simulink library "libbha_parameters"  (R2015b)
settings: Solver=FixedStepDiscrete  StartTime=0.0  StopTime=Inf  FixedStep=0.004  RelTol=1e-3
PostLoadFcn:
  | , if any(exist('dsrtsu_mdlpostloadfcn', 'file') == [2, 3, 6]), try dsrtsu_mdlpostloadfcn('Execute', bdroot); catch fprintf('Error in PostLoadFcn (dsrtsu_mdlpostloadfcn) for model "%s":\n %s\n', bdroot, lasterr); end, end,
undefined symbols (not defined in the file or in its folder): BHA, CONST
libraries: libbha_kinematic x12
(part 1 of 2)
settings Model: DSRTSU_INTERNAL_RTI_VER=470  DSRTSU_INTERNAL_RTI_TYPE=rti1005  DSRTSU_INTERNAL_RTIFPGA=60  Creator=Falkenhahn  LastModifiedBy=fav
settings DataIOCC: SaveFormat=Array
settings OptimizationCC: BlockReduction=off  OptimizeBlockIOStorage=off  BufferReuse=off  GlobalBufferReuse=off  ExpressionFolding=off  LocalBlockOutputs=off
settings DebuggingCC: UnderspecifiedInitializationDetection=Classic  MergeDetectMultiDrivingBlocksExec=none  SolverPrmCheckMsg=warning
settings HardwareCC: ProdBitPerPointer=32  ProdLargestAtomicFloat=None  ProdEndianess=BigEndian  ProdWordSize=32  ProdHWDeviceType=Generic->Custom  TargetIntDivRoundTo=Zero  TargetEndianess=BigEndian  TargetHWDeviceType=Generic->Custom
settings RTWCC: SystemTargetFile=rti1007.tlc  MakeCommand=make_rti  TemplateMakefile=rti1007.tmf  Description=dSPACE DS1007 Hardware Platform
settings STFCustomTargetCC: ParMdlRefBuildCompliant=on  ConcurrentExecutionCompliant=off  MatFileLogging=on  SystemTargetFile=rti1007.tlc
settings GRTTargetCC: CompOptLevelCompliant=off  ConcurrentExecutionCompliant=off  GeneratePreprocessorConditionals=Disable all  CombineOutputUpdateFcns=off  GRTInterface=on  UseToolchainInfoCompliant=off  ExtModeMexFile=noextcomm
settings ConfigComp: CovModelRefEnable=Off

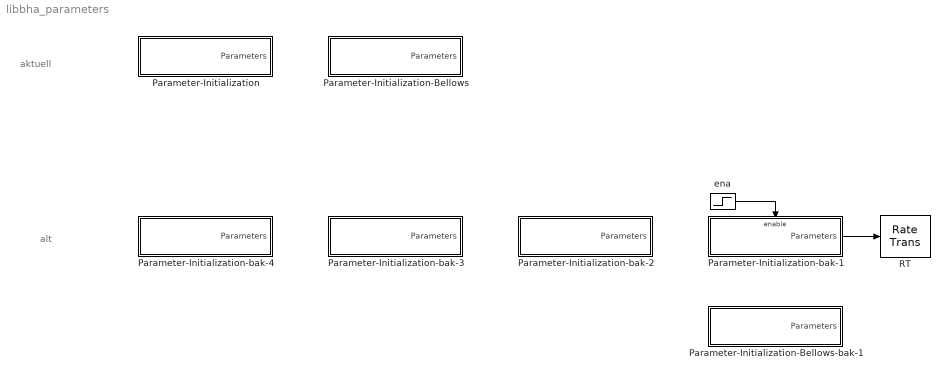
== system libbha_parameters ==
  note: aktuell
  note: alt
  Parameter-Initialization : Subsystem  mask{bha_var_choice=BHA, tA=CONST.tA}
      mask prompts: bha_var_choice "BHA-Parameter"; tA "sample time"
      mask init:
      | if bha_var_choice == 1 % BHA
      |     bha_var = evalin('base','BHA');
      | elseif bha_var_choice == 2 % BHASIM
      |     bha_var = evalin('base','BHASIM');
      | else % default: BHA
      |     bha_var = evalin('base','BHA');
      | end
      settings: AttributesFormatString=|
      | BHA-Variable: %<bha_var_choice>
      | sample time: %<tA>
      mask TypeOptions bha_var_choice: BHA | BHASIM
  Parameter-Initialization-Bellows : Subsystem  mask{bha_var_choice=BHA, tA=CONST.tA}
      mask prompts: bha_var_choice "BHA-Parameter"; tA "sample time"
      mask init:
      | if bha_var_choice == 1 % BHA
      |     bha_var = evalin('base','BHA');
      | elseif bha_var_choice == 2 % BHASIM
      |     bha_var = evalin('base','BHASIM');
      | else % default: BHA
      |     bha_var = evalin('base','BHA');
      | end
      settings: AttributesFormatString=|
      | BHA-Variable: %<bha_var_choice>\nsample time: %<tA>
      | (ohne Manipulatordaten)
      mask TypeOptions bha_var_choice: BHA | BHASIM
  Parameter-Initialization-Bellows-bak-1 : Subsystem  mask{bha_var_choice=BHA, tA=CONST.tA}
      mask prompts: bha_var_choice "BHA-Parameter"; tA "sample time"
      mask init:
      | if bha_var_choice == 1 % BHA
      |     bha_var = evalin('base','BHA');
      | elseif bha_var_choice == 2 % BHASIM
      |     bha_var = evalin('base','BHASIM');
      | else % default: BHA
      |     bha_var = evalin('base','BHA');
      | end
      settings: AttributesFormatString=|
      | BHA-Variable: %<bha_var_choice>\nsample time: %<tA>
      | (ohne Manipulatordaten)
      mask TypeOptions bha_var_choice: BHA | BHASIM
  Parameter-Initialization-bak-1 : Subsystem  mask{bha_var_choice=BHA}
      mask prompts: bha_var_choice "BHA-Parameter"
      mask init:
      | if bha_var_choice == 1 % BHA
      |     bha_var = evalin('base','BHA');
      | elseif bha_var_choice == 2 % BHASIM
      |     bha_var = evalin('base','BHASIM');
      | else % default: BHA
      |     bha_var = evalin('base','BHA');
      | end
      settings: AttributesFormatString=BHA-Variable: %<bha_var_choice>
      mask TypeOptions bha_var_choice: BHA | BHASIM
  Parameter-Initialization-bak-2 : Subsystem  mask{bha_var_choice=BHA, tA=CONST.tA}
      mask prompts: bha_var_choice "BHA-Parameter"; tA "sample time"
      mask init:
      | if bha_var_choice == 1 % BHA
      |     bha_var = evalin('base','BHA');
      | elseif bha_var_choice == 2 % BHASIM
      |     bha_var = evalin('base','BHASIM');
      | else % default: BHA
      |     bha_var = evalin('base','BHA');
      | end
      settings: AttributesFormatString=BHA-Variable: %<bha_var_choice>\nsample time: %<tA>
      mask TypeOptions bha_var_choice: BHA | BHASIM
  Parameter-Initialization-bak-3 : Subsystem  mask{bha_var_choice=BHA, tA=CONST.tA}
      mask prompts: bha_var_choice "BHA-Parameter"; tA "sample time"
      mask init:
      | if bha_var_choice == 1 % BHA
      |     bha_var = evalin('base','BHA');
      | elseif bha_var_choice == 2 % BHASIM
      |     bha_var = evalin('base','BHASIM');
      | else % default: BHA
      |     bha_var = evalin('base','BHA');
      | end
      settings: AttributesFormatString=BHA-Variable: %<bha_var_choice>\nsample time: %<tA>
      mask TypeOptions bha_var_choice: BHA | BHASIM
  Parameter-Initialization-bak-4 : Subsystem  mask{bha_var_choice=BHA, tA=CONST.tA}
      mask prompts: bha_var_choice "BHA-Parameter"; tA "sample time"
      mask init:
      | if bha_var_choice == 1 % BHA
      |     bha_var = evalin('base','BHA');
      | elseif bha_var_choice == 2 % BHASIM
      |     bha_var = evalin('base','BHASIM');
      | else % default: BHA
      |     bha_var = evalin('base','BHA');
      | end
      settings: AttributesFormatString=BHA-Variable: %<bha_var_choice>\nsample time: %<tA>
      mask TypeOptions bha_var_choice: BHA | BHASIM
  RT : RateTransition  Deterministic=off  OutPortSampleTime=CTRL.tA.obsv_pr
      settings: AttributesFormatString=%<OutPortSampleTime>
  ena : Step  Time=2*CONST.tA  Before=1  After=0  SampleTime=CONST.tA
  wires:
  ena/1 -> Parameter-Initialization-bak-1/Enable
  Parameter-Initialization-bak-1/1(Parameters) -> RT/1

== system libbha_parameters/Parameter-Initialization ==
  Calculate Parameters Once : Subsystem
  ena : Step  Time=2*tA  Before=1  After=0  SampleTime=tA
  Parameters : Outport  SourceOfInitialOutputValue=Input signal
  wires:
  Calculate Parameters Once/1(Parameters) -> Parameters/1
  ena/1 -> Calculate Parameters Once/Enable

== system libbha_parameters/Parameter-Initialization-Bellows ==
  Calculate Parameters Once : Subsystem
  ena : Step  Time=2*tA  Before=1  After=0  SampleTime=tA
  Parameters : Outport  SourceOfInitialOutputValue=Input signal
  wires:
  ena/1 -> Calculate Parameters Once/Enable
  Calculate Parameters Once/1(Parameters) -> Parameters/1

== system libbha_parameters/Parameter-Initialization-Bellows-bak-1 ==
  Calculate Parameters Once : Subsystem
  ena : Step  Time=2*tA  Before=1  After=0  SampleTime=tA
  Parameters : Outport  SourceOfInitialOutputValue=Input signal
  wires:
  Calculate Parameters Once/1(Parameters) -> Parameters/1
  ena/1 -> Calculate Parameters Once/Enable

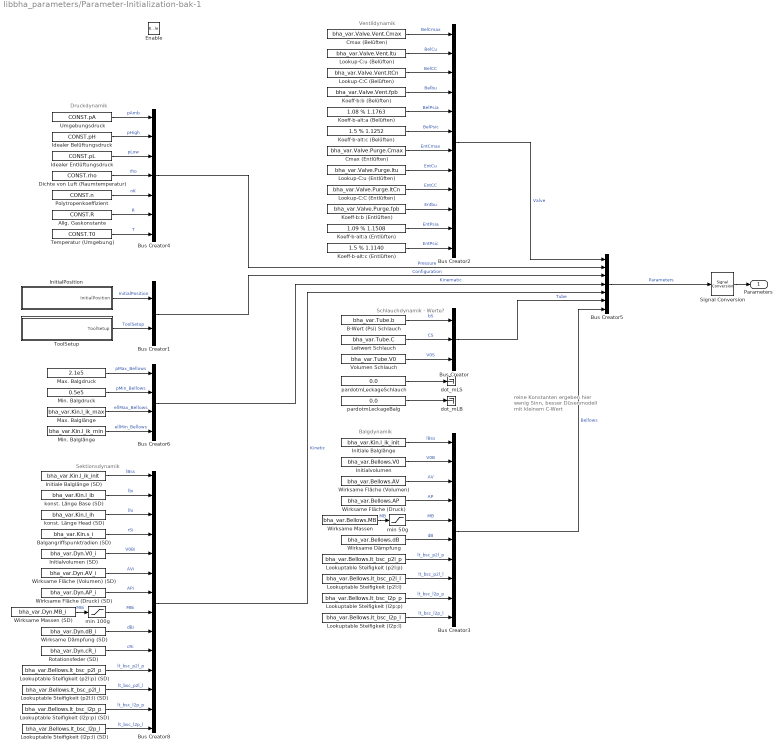
== system libbha_parameters/Parameter-Initialization-bak-1 ==
  note: Sektionsdynamik
  note: Ventildynamik
  note: Druckdynamik
  note: Balgdynamik
  note: Schlauchdynamik - Werte?
  note: reine Konstanten ergeben
      | hier wenig Sinn, besser
      | Düsenmodell mit kleinem C-Wert
  Enable : EnablePort  PropagateVarSize=During execution
  Allg. Gaskonstante : Constant  Value=CONST.R
  B-Wert (Psi) Schlauch : Constant  Value=bha_var.Tube.b
  Balgangriffspunktradien (SD) : Constant  Value=bha_var.Kin.s_i
  Bus Creator1 : BusCreator  Inputs=2
  Bus Creator3 : BusCreator  Inputs=10
  Bus Creator4 : BusCreator  Inputs=7
  Bus Creator6 : BusCreator  Inputs=4
  Bus Creator8 : BusCreator  Inputs=14
  Bus Creator : BusCreator  Inputs=3
  Bus Creator2 : BusCreator  Inputs=12
  Bus Creator5 : BusCreator  Inputs=7
  Cmax (Belüften) : Constant  Value=bha_var.Valve.Vent.Cmax
  Cmax (Entlüften) : Constant  Value=bha_var.Valve.Purge.Cmax
  Dichte von Luft (Raumtemperatur) : Constant  Value=CONST.rho
  Idealer Belüftungsdruck : Constant  Value=CONST.pH
  Idealer Entlüftungsdruck : Constant  Value=CONST.pL
  InitialPosition : Subsystem
  Initiale Balglänge : Constant  Value=bha_var.Kin.l_ik_init
  Initiale Balglänge (SD) : Constant  Value=bha_var.Kin.l_ik_init
  Initialvolumen : Constant  Value=bha_var.Bellows.V0
  Initialvolumen (SD) : Constant  Value=bha_var.Dyn.V0_i
  Koeff-b-alt:a (Belüften) : Constant  Value=1.08 % 1.1763
  Koeff-b-alt:a (Entlüften) : Constant  Value=1.09 % 1.1508
  Koeff-b-alt:c (Belüften) : Constant  Value=1.5 % 1.1252
  Koeff-b-alt:c (Entlüften) : Constant  Value=1.5 % 1.1140
  Koeff-b:b (Belüften) : Constant  Value=bha_var.Valve.Vent.fpb
  Koeff-b:b (Entlüften) : Constant  Value=bha_var.Valve.Purge.fpb
  Leitwert Schlauch : Constant  Value=bha_var.Tube.C
  Lookup-C:C (Belüften) : Constant  Value=bha_var.Valve.Vent.ltCn
  Lookup-C:C (Entlüften) : Constant  Value=bha_var.Valve.Purge.ltCn
  Lookup-C:u (Belüften) : Constant  Value=bha_var.Valve.Vent.ltu
  Lookup-C:u (Entlüften) : Constant  Value=bha_var.Valve.Purge.ltu
  Lookuptable Steifigkeit (l2p:l) : Constant  Value=bha_var.Bellows.lt_bsc_l2p_l
  Lookuptable Steifigkeit (l2p:l) (SD) : Constant  Value=bha_var.Bellows.lt_bsc_l2p_l
  Lookuptable Steifigkeit (l2p:p) : Constant  Value=bha_var.Bellows.lt_bsc_l2p_p
  Lookuptable Steifigkeit (l2p:p) (SD) : Constant  Value=bha_var.Bellows.lt_bsc_l2p_p
  Lookuptable Steifigkeit (p2l:l) : Constant  Value=bha_var.Bellows.lt_bsc_p2l_l
  Lookuptable Steifigkeit (p2l:l) (SD) : Constant  Value=bha_var.Bellows.lt_bsc_p2l_l
  Lookuptable Steifigkeit (p2l:p) : Constant  Value=bha_var.Bellows.lt_bsc_p2l_p
  Lookuptable Steifigkeit (p2l:p) (SD) : Constant  Value=bha_var.Bellows.lt_bsc_p2l_p
  Max. Balgdruck : Constant  Value=2.1e5
  Max. Balglänge : Constant  Value=bha_var.Kin.l_ik_max
  Min. Balgdruck : Constant  Value=0.5e5
  Min. Balglänge : Constant  Value=bha_var.Kin.l_ik_min
  Polytropenkoeffizient : Constant  Value=CONST.n
  Rotationsfeder (SD) : Constant  Value=bha_var.Dyn.cR_i
  Signal Conversion : SignalConversion
  Temperatur (Umgebung) : Constant  Value=CONST.T0
  ToolSetup : Subsystem
  Umgebungsdruck : Constant  Value=CONST.pA
  Volumen Schlauch : Constant  Value=bha_var.Tube.V0
  Wirksame Dämpfung : Constant  Value=bha_var.Bellows.dB
  Wirksame Dämpfung (SD) : Constant  Value=bha_var.Dyn.dB_i
  Wirksame Fläche (Druck) : Constant  Value=bha_var.Bellows.AP
  Wirksame Fläche (Druck) (SD) : Constant  Value=bha_var.Dyn.AP_i
  Wirksame Fläche (Volumen) : Constant  Value=bha_var.Bellows.AV
  Wirksame Fläche (Volumen) (SD) : Constant  Value=bha_var.Dyn.AV_i
  Wirksame Massen : Constant  Value=bha_var.Bellows.MB
  Wirksame Massen (SD) : Constant  Value=bha_var.Dyn.MB_i
  dot_mLB : Terminator
  dot_mLS : Terminator
  konst. Länge Base (SD) : Constant  Value=bha_var.Kin.l_ib
  konst. Länge Head (SD) : Constant  Value=bha_var.Kin.l_ih
  min 100g : Saturate  UpperLimit=inf  LowerLimit=0.1
  min 50g : Saturate  UpperLimit=inf  LowerLimit=0.1
  pardotmLeckageBalg : Constant  Value=0.0
  pardotmLeckageSchlauch : Constant  Value=0.0
  Parameters : Outport  SourceOfInitialOutputValue=Input signal
  wires:
  Signal Conversion/1 -> Parameters/1
  Koeff-b-alt:c (Entlüften)/1 -> Bus Creator2/12  "EntPsic"
  Koeff-b-alt:c (Belüften)/1 -> Bus Creator2/6  "BelPsic"
  Koeff-b-alt:a (Belüften)/1 -> Bus Creator2/5  "BelPsia"
  Koeff-b-alt:a (Entlüften)/1 -> Bus Creator2/11  "EntPsia"
  Bus Creator4/1 -> Bus Creator5/2  "Pressure"
  Umgebungsdruck/1 -> Bus Creator4/1  "pAmb"
  Idealer Belüftungsdruck/1 -> Bus Creator4/2  "pHigh"
  Bus Creator5/1 -> Signal Conversion/1  "Parameters"
  Bus Creator1/1 -> Bus Creator5/3  "Configuration"
  InitialPosition/1(InitialPosition) -> Bus Creator1/1  "InitialPosition"
  Idealer Entlüftungsdruck/1 -> Bus Creator4/3  "pLow"
  ToolSetup/1(ToolSetup) -> Bus Creator1/2  "ToolSetup"
  Dichte von Luft (Raumtemperatur)/1 -> Bus Creator4/4  "rho"
  Polytropenkoeffizient/1 -> Bus Creator4/5  "nK"
  Allg. Gaskonstante/1 -> Bus Creator4/6  "R"
  Temperatur (Umgebung)/1 -> Bus Creator4/7  "T"
  Bus Creator2/1 -> Bus Creator5/1  "Valve"
  Lookup-C:u (Belüften)/1 -> Bus Creator2/2  "BelCu"
  Cmax (Belüften)/1 -> Bus Creator2/1  "BelCmax"
  Lookup-C:C (Belüften)/1 -> Bus Creator2/3  "BelCC"
  Cmax (Entlüften)/1 -> Bus Creator2/7  "EntCmax"
  Lookup-C:u (Entlüften)/1 -> Bus Creator2/8  "EntCu"
  Lookup-C:C (Entlüften)/1 -> Bus Creator2/9  "EntCC"
  Koeff-b:b (Belüften)/1 -> Bus Creator2/4  "Belbu"
  Koeff-b:b (Entlüften)/1 -> Bus Creator2/10  "Entbu"
  min 50g/1 -> Bus Creator3/5  "MB"
  Wirksame Dämpfung/1 -> Bus Creator3/6  "dB"
  Wirksame Fläche (Volumen)/1 -> Bus Creator3/3  "AV"
  Initialvolumen/1 -> Bus Creator3/2  "V0B"
  Initiale Balglänge/1 -> Bus Creator3/1  "lBss"
  Wirksame Fläche (Druck)/1 -> Bus Creator3/4  "AP"
  B-Wert (Psi) Schlauch/1 -> Bus Creator/1  "bS"
  Volumen Schlauch/1 -> Bus Creator/3  "V0S"
  Leitwert Schlauch/1 -> Bus Creator/2  "CS"
  Bus Creator/1 -> Bus Creator5/6  "Tube"
  Bus Creator3/1 -> Bus Creator5/7  "Bellows"
  Bus Creator6/1 -> Bus Creator5/4  "Kinematic"
  pardotmLeckageSchlauch/1 -> dot_mLS/1
  pardotmLeckageBalg/1 -> dot_mLB/1
  Max. Balgdruck/1 -> Bus Creator6/1  "pMax_Bellows"
  Bus Creator8/1 -> Bus Creator5/5  "Kinetic"
  min 100g/1 -> Bus Creator8/8  "MBi"
  Initiale Balglänge (SD)/1 -> Bus Creator8/1  "lBss"
  Initialvolumen (SD)/1 -> Bus Creator8/5  "V0Bi"
  Wirksame Dämpfung (SD)/1 -> Bus Creator8/9  "dBi"
  Wirksame Fläche (Druck) (SD)/1 -> Bus Creator8/7  "APi"
  Wirksame Fläche (Volumen) (SD)/1 -> Bus Creator8/6  "AVi"
  Rotationsfeder (SD)/1 -> Bus Creator8/10  "cRi"
  Balgangriffspunktradien (SD)/1 -> Bus Creator8/4  "rSi"
  konst. Länge Base (SD)/1 -> Bus Creator8/2  "lbi"
  konst. Länge Head (SD)/1 -> Bus Creator8/3  "lhi"
  Min. Balgdruck/1 -> Bus Creator6/2  "pMin_Bellows"
  Min. Balglänge/1 -> Bus Creator6/4  "ellMin_Bellows"
  Max. Balglänge/1 -> Bus Creator6/3  "ellMax_Bellows"
  Lookuptable Steifigkeit (l2p:p)/1 -> Bus Creator3/9  "lt_bsc_l2p_p"
  Lookuptable Steifigkeit (l2p:l)/1 -> Bus Creator3/10  "lt_bsc_l2p_l"
  Lookuptable Steifigkeit (p2l:p)/1 -> Bus Creator3/7  "lt_bsc_p2l_p"
  Lookuptable Steifigkeit (p2l:l)/1 -> Bus Creator3/8  "lt_bsc_p2l_l"
  Lookuptable Steifigkeit (l2p:p) (SD)/1 -> Bus Creator8/13  "lt_bsc_l2p_p"
  Lookuptable Steifigkeit (l2p:l) (SD)/1 -> Bus Creator8/14  "lt_bsc_l2p_l"
  Lookuptable Steifigkeit (p2l:l) (SD)/1 -> Bus Creator8/12  "lt_bsc_p2l_l"
  Lookuptable Steifigkeit (p2l:p) (SD)/1 -> Bus Creator8/11  "lt_bsc_p2l_p"
  Wirksame Massen (SD)/1 -> min 100g/1  "MBi"
  Wirksame Massen/1 -> min 50g/1  "MB"

== system libbha_parameters/Parameter-Initialization-bak-2 ==
  Calculate Parameters Once : Subsystem
  ena : Step  Time=2*tA  Before=1  After=0  SampleTime=tA
  Parameters : Outport  SourceOfInitialOutputValue=Input signal
  wires:
  ena/1 -> Calculate Parameters Once/Enable
  Calculate Parameters Once/1(Parameters) -> Parameters/1

== system libbha_parameters/Parameter-Initialization-bak-3 ==
  Calculate Parameters Once : Subsystem
  ena : Step  Time=2*tA  Before=1  After=0  SampleTime=tA
  Parameters : Outport  SourceOfInitialOutputValue=Input signal
  wires:
  ena/1 -> Calculate Parameters Once/Enable
  Calculate Parameters Once/1(Parameters) -> Parameters/1

== system libbha_parameters/Parameter-Initialization-bak-4 ==
  Calculate Parameters Once : Subsystem
  ena : Step  Time=2*tA  Before=1  After=0  SampleTime=tA
  Parameters : Outport  SourceOfInitialOutputValue=Input signal
  wires:
  ena/1 -> Calculate Parameters Once/Enable
  Calculate Parameters Once/1(Parameters) -> Parameters/1

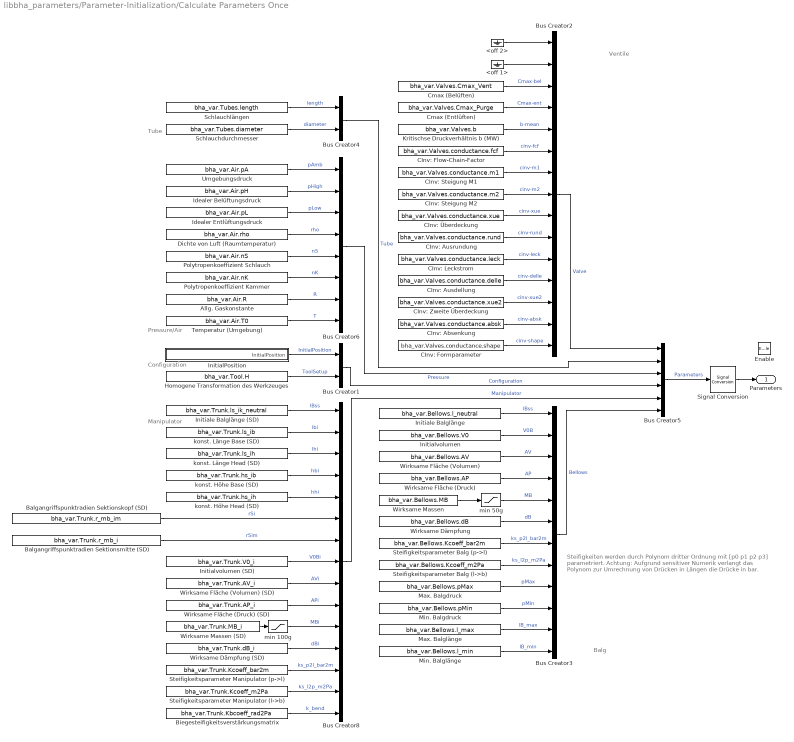
== system libbha_parameters/Parameter-Initialization/Calculate Parameters Once ==
  note: Steifigkeiten werden durch Polynom dritter Ordnung mit [p0 p1 p2 p3]
      | parametriert. Achtung: Aufgrund sensitiver Numerik verlangt das Polynom
      | zur Umrechnung von Drücken in Längen die Drücke in bar.
  note: Balg
  note: Ventile
  note: Manipulator
  note: Configuration
  note: Pressure/Air
  note: Tube
  Enable : EnablePort  PropagateVarSize=During execution
  <off 1> : Ground
  <off 2> : Ground
  Allg. Gaskonstante : Constant  Value=bha_var.Air.R
  Balgangriffspunktradien Sektionskopf (SD) : Constant  Value=bha_var.Trunk.r_mb_im
      settings: AttributesFormatString=|
      | Radien Manipulator-Balg
      | r_mb_im: am Sektionskopf
      | r_mb_i:    an Sektionsmitte
      | r_mb_i0:  an Sektionsfuß
  Balgangriffspunktradien Sektionsmitte (SD) : Constant  Value=bha_var.Trunk.r_mb_i
      settings: AttributesFormatString=|
      | Radien Manipulator-Balg
      | r_mb_im: am Sektionskopf
      | r_mb_i:    an Sektionsmitte
      | r_mb_i0:  an Sektionsfuß
  Biegesteifigkeitsverstärkungsmatrix : Constant  Value=bha_var.Trunk.Kbcoeff_rad2Pa
  Bus Creator1 : BusCreator  Inputs=2
  Bus Creator3 : BusCreator  Inputs=12
  Bus Creator4 : BusCreator  Inputs=2
  Bus Creator6 : BusCreator  Inputs=8
  Bus Creator8 : BusCreator  Inputs=15
  Bus Creator2 : BusCreator  Inputs=15
  Bus Creator5 : BusCreator  Inputs=6
  CInv: Absenkung : Constant  Value=bha_var.Valves.conductance.absk
  CInv: Ausdellung : Constant  Value=bha_var.Valves.conductance.delle
  CInv: Ausrundung : Constant  Value=bha_var.Valves.conductance.rund
  CInv: Flow-Chain-Factor : Constant  Value=bha_var.Valves.conductance.fcf
  CInv: Formparameter : Constant  Value=bha_var.Valves.conductance.shape
  CInv: Leckstrom : Constant  Value=bha_var.Valves.conductance.leck
  CInv: Steigung M1 : Constant  Value=bha_var.Valves.conductance.m1
  CInv: Steigung M2 : Constant  Value=bha_var.Valves.conductance.m2
  CInv: Zweite Überdeckung : Constant  Value=bha_var.Valves.conductance.xue2
  CInv: Überdeckung : Constant  Value=bha_var.Valves.conductance.xue
  Cmax (Belüften) : Constant  Value=bha_var.Valves.Cmax_Vent
  Cmax (Entlüften) : Constant  Value=bha_var.Valves.Cmax_Purge
  Dichte von Luft (Raumtemperatur) : Constant  Value=bha_var.Air.rho
  Homogene Transformation des Werkzeuges : Constant  Value=bha_var.Tool.H
  Idealer Belüftungsdruck : Constant  Value=bha_var.Air.pH
  Idealer Entlüftungsdruck : Constant  Value=bha_var.Air.pL
  InitialPosition : Subsystem
  Initiale Balglänge : Constant  Value=bha_var.Bellows.l_neutral
  Initiale Balglänge (SD) : Constant  Value=bha_var.Trunk.ls_ik_neutral
  Initialvolumen : Constant  Value=bha_var.Bellows.V0
  Initialvolumen (SD) : Constant  Value=bha_var.Trunk.V0_i
  Kritischse Druckverhältnis b (MW) : Constant  Value=bha_var.Valves.b
  Max. Balgdruck : Constant  Value=bha_var.Bellows.pMax
  Max. Balglänge : Constant  Value=bha_var.Bellows.l_max
  Min. Balgdruck : Constant  Value=bha_var.Bellows.pMin
  Min. Balglänge : Constant  Value=bha_var.Bellows.l_min
  Polytropenkoeffizient Kammer : Constant  Value=bha_var.Air.nK
  Polytropenkoeffizient Schlauch : Constant  Value=bha_var.Air.nS
  Schlauchdurchmesser : Constant  Value=bha_var.Tubes.diameter
  Schlauchlängen : Constant  Value=bha_var.Tubes.length
  Signal Conversion : SignalConversion
  Steifigkeitsparameter Balg (l->b) : Constant  Value=bha_var.Bellows.Kcoeff_m2Pa
  Steifigkeitsparameter Balg (p->l) : Constant  Value=bha_var.Bellows.Kcoeff_bar2m
  Steifigkeitsparameter Manipulator (l->b) : Constant  Value=bha_var.Trunk.Kcoeff_m2Pa
  Steifigkeitsparameter Manipulator (p->l) : Constant  Value=bha_var.Trunk.Kcoeff_bar2m
  Temperatur (Umgebung) : Constant  Value=bha_var.Air.T0
  Umgebungsdruck : Constant  Value=bha_var.Air.pA
  Wirksame Dämpfung : Constant  Value=bha_var.Bellows.dB
  Wirksame Dämpfung (SD) : Constant  Value=bha_var.Trunk.dB_i
  Wirksame Fläche (Druck) : Constant  Value=bha_var.Bellows.AP
  Wirksame Fläche (Druck) (SD) : Constant  Value=bha_var.Trunk.AP_i
  Wirksame Fläche (Volumen) : Constant  Value=bha_var.Bellows.AV
  Wirksame Fläche (Volumen) (SD) : Constant  Value=bha_var.Trunk.AV_i
  Wirksame Massen : Constant  Value=bha_var.Bellows.MB
  Wirksame Massen (SD) : Constant  Value=bha_var.Trunk.MB_i
  konst. Höhe Base (SD) : Constant  Value=bha_var.Trunk.hs_ib
  konst. Höhe Head (SD) : Constant  Value=bha_var.Trunk.hs_ih
  konst. Länge Base (SD) : Constant  Value=bha_var.Trunk.ls_ib
  konst. Länge Head (SD) : Constant  Value=bha_var.Trunk.ls_ih
  min 100g : Saturate  UpperLimit=inf  LowerLimit=0.1
  min 50g : Saturate  UpperLimit=inf  LowerLimit=0.1
  Parameters : Outport
  wires:
  Schlauchdurchmesser/1 -> Bus Creator4/2  "diameter"
  Schlauchlängen/1 -> Bus Creator4/1  "length"
  Min. Balglänge/1 -> Bus Creator3/12  "lB_min"
  Max. Balglänge/1 -> Bus Creator3/11  "lB_max"
  Min. Balgdruck/1 -> Bus Creator3/10  "pMin"
  Max. Balgdruck/1 -> Bus Creator3/9  "pMax"
  CInv: Flow-Chain-Factor/1 -> Bus Creator2/6  "cinv-fcf"
  CInv: Steigung M1/1 -> Bus Creator2/7  "cinv-m1"
  CInv: Steigung M2/1 -> Bus Creator2/8  "cinv-m2"
  CInv: Überdeckung/1 -> Bus Creator2/9  "cinv-xue"
  CInv: Ausrundung/1 -> Bus Creator2/10  "cinv-rund"
  CInv: Leckstrom/1 -> Bus Creator2/11  "cinv-leck"
  Cmax (Entlüften)/1 -> Bus Creator2/4  "Cmax-ent"
  Cmax (Belüften)/1 -> Bus Creator2/3  "Cmax-bel"
  Idealer Belüftungsdruck/1 -> Bus Creator6/2  "pHigh"
  Signal Conversion/1 -> Parameters/1
  Bus Creator1/1 -> Bus Creator5/4  "Configuration"
  Initiale Balglänge (SD)/1 -> Bus Creator8/1  "lBss"
  Bus Creator6/1 -> Bus Creator5/3  "Pressure"
  Steifigkeitsparameter Balg (l->b)/1 -> Bus Creator3/8  "ks_l2p_m2Pa"
  InitialPosition/1(InitialPosition) -> Bus Creator1/1  "InitialPosition"
  Allg. Gaskonstante/1 -> Bus Creator6/7  "R"
  Polytropenkoeffizient Kammer/1 -> Bus Creator6/6  "nK"
  Bus Creator2/1 -> Bus Creator5/1  "Valve"
  Wirksame Fläche (Volumen)/1 -> Bus Creator3/3  "AV"
  Idealer Entlüftungsdruck/1 -> Bus Creator6/3  "pLow"
  Temperatur (Umgebung)/1 -> Bus Creator6/8  "T"
  Dichte von Luft (Raumtemperatur)/1 -> Bus Creator6/4  "rho"
  Wirksame Dämpfung/1 -> Bus Creator3/6  "dB"
  min 50g/1 -> Bus Creator3/5  "MB"
  konst. Länge Base (SD)/1 -> Bus Creator8/2  "lbi"
  konst. Länge Head (SD)/1 -> Bus Creator8/3  "lhi"
  Steifigkeitsparameter Balg (p->l)/1 -> Bus Creator3/7  "ks_p2l_bar2m"
  Initialvolumen/1 -> Bus Creator3/2  "V0B"
  Homogene Transformation des Werkzeuges/1 -> Bus Creator1/2  "ToolSetup"
  Bus Creator3/1 -> Bus Creator5/6  "Bellows"
  Bus Creator8/1 -> Bus Creator5/5  "Manipulator"
  Wirksame Fläche (Druck)/1 -> Bus Creator3/4  "AP"
  Initiale Balglänge/1 -> Bus Creator3/1  "lBss"
  Umgebungsdruck/1 -> Bus Creator6/1  "pAmb"
  Wirksame Massen (SD)/1 -> min 100g/1
  Wirksame Massen/1 -> min 50g/1
  Bus Creator5/1 -> Signal Conversion/1  "Parameters"
  Bus Creator4/1 -> Bus Creator5/2  "Tube"
  Kritischse Druckverhältnis b (MW)/1 -> Bus Creator2/5  "b-mean"
  CInv: Absenkung/1 -> Bus Creator2/14  "cinv-absk"
  CInv: Formparameter/1 -> Bus Creator2/15  "cinv-shape"
  CInv: Ausdellung/1 -> Bus Creator2/12  "cinv-delle"
  CInv: Zweite Überdeckung/1 -> Bus Creator2/13  "cinv-xue2"
  <off 1>/1 -> Bus Creator2/2
  <off 2>/1 -> Bus Creator2/1
  konst. Höhe Base (SD)/1 -> Bus Creator8/4  "hbi"
  konst. Höhe Head (SD)/1 -> Bus Creator8/5  "hhi"
  Balgangriffspunktradien Sektionskopf (SD)/1 -> Bus Creator8/6  "rSi"
  Balgangriffspunktradien Sektionsmitte (SD)/1 -> Bus Creator8/7  "rSim"
  Initialvolumen (SD)/1 -> Bus Creator8/8  "V0Bi"
  Steifigkeitsparameter Manipulator (p->l)/1 -> Bus Creator8/13  "ks_p2l_bar2m"
  Wirksame Dämpfung (SD)/1 -> Bus Creator8/12  "dBi"
  min 100g/1 -> Bus Creator8/11  "MBi"
  Steifigkeitsparameter Manipulator (l->b)/1 -> Bus Creator8/14  "ks_l2p_m2Pa"
  Wirksame Fläche (Druck) (SD)/1 -> Bus Creator8/10  "APi"
  Wirksame Fläche (Volumen) (SD)/1 -> Bus Creator8/9  "AVi"
  Biegesteifigkeitsverstärkungsmatrix/1 -> Bus Creator8/15  "k_bend"
  Polytropenkoeffizient Schlauch/1 -> Bus Creator6/5  "nS"

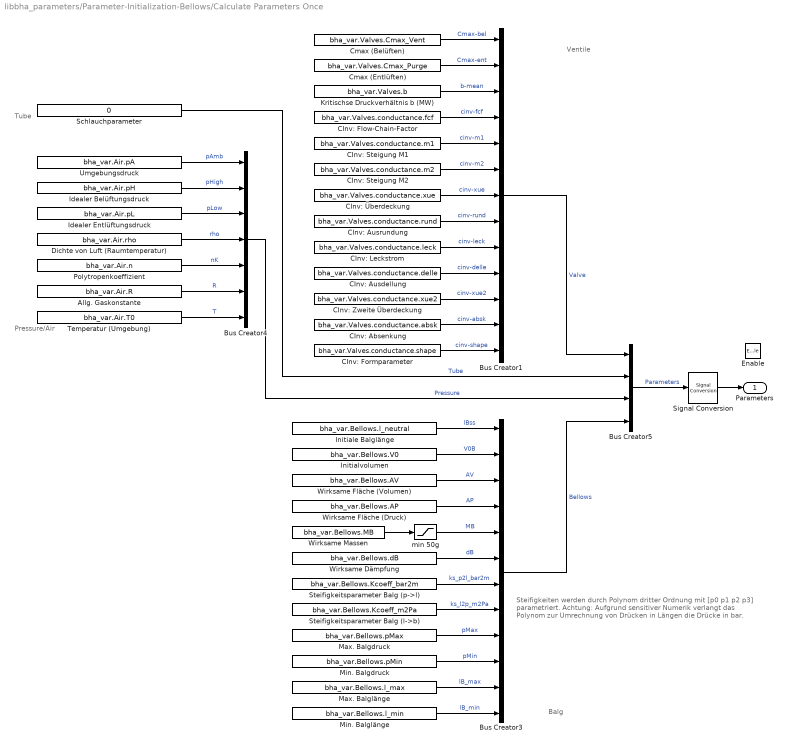
== system libbha_parameters/Parameter-Initialization-Bellows/Calculate Parameters Once ==
  note: Tube
  note: Pressure/Air
  note: Balg
  note: Steifigkeiten werden durch Polynom dritter Ordnung mit [p0 p1 p2 p3]
      | parametriert. Achtung: Aufgrund sensitiver Numerik verlangt das Polynom
      | zur Umrechnung von Drücken in Längen die Drücke in bar.
  note: Ventile
  Enable : EnablePort  PropagateVarSize=During execution
  Allg. Gaskonstante : Constant  Value=bha_var.Air.R
  Bus Creator3 : BusCreator  Inputs=12
  Bus Creator4 : BusCreator  Inputs=7
  Bus Creator1 : BusCreator  Inputs=13
  Bus Creator5 : BusCreator  Inputs=4
  CInv: Absenkung : Constant  Value=bha_var.Valves.conductance.absk
  CInv: Ausdellung : Constant  Value=bha_var.Valves.conductance.delle
  CInv: Ausrundung : Constant  Value=bha_var.Valves.conductance.rund
  CInv: Flow-Chain-Factor : Constant  Value=bha_var.Valves.conductance.fcf
  CInv: Formparameter : Constant  Value=bha_var.Valves.conductance.shape
  CInv: Leckstrom : Constant  Value=bha_var.Valves.conductance.leck
  CInv: Steigung M1 : Constant  Value=bha_var.Valves.conductance.m1
  CInv: Steigung M2 : Constant  Value=bha_var.Valves.conductance.m2
  CInv: Zweite Überdeckung : Constant  Value=bha_var.Valves.conductance.xue2
  CInv: Überdeckung : Constant  Value=bha_var.Valves.conductance.xue
  Cmax (Belüften) : Constant  Value=bha_var.Valves.Cmax_Vent
  Cmax (Entlüften) : Constant  Value=bha_var.Valves.Cmax_Purge
  Dichte von Luft (Raumtemperatur) : Constant  Value=bha_var.Air.rho
  Idealer Belüftungsdruck : Constant  Value=bha_var.Air.pH
  Idealer Entlüftungsdruck : Constant  Value=bha_var.Air.pL
  Initiale Balglänge : Constant  Value=bha_var.Bellows.l_neutral
  Initialvolumen : Constant  Value=bha_var.Bellows.V0
  Kritischse Druckverhältnis b (MW) : Constant  Value=bha_var.Valves.b
  Max. Balgdruck : Constant  Value=bha_var.Bellows.pMax
  Max. Balglänge : Constant  Value=bha_var.Bellows.l_max
  Min. Balgdruck : Constant  Value=bha_var.Bellows.pMin
  Min. Balglänge : Constant  Value=bha_var.Bellows.l_min
  Polytropenkoeffizient : Constant  Value=bha_var.Air.n
  Schlauchparameter : Constant  Value=0
  Signal Conversion : SignalConversion
  Steifigkeitsparameter Balg (l->b) : Constant  Value=bha_var.Bellows.Kcoeff_m2Pa
  Steifigkeitsparameter Balg (p->l) : Constant  Value=bha_var.Bellows.Kcoeff_bar2m
  Temperatur (Umgebung) : Constant  Value=bha_var.Air.T0
  Umgebungsdruck : Constant  Value=bha_var.Air.pA
  Wirksame Dämpfung : Constant  Value=bha_var.Bellows.dB
  Wirksame Fläche (Druck) : Constant  Value=bha_var.Bellows.AP
  Wirksame Fläche (Volumen) : Constant  Value=bha_var.Bellows.AV
  Wirksame Massen : Constant  Value=bha_var.Bellows.MB
  min 50g : Saturate  UpperLimit=inf  LowerLimit=0.1
  Parameters : Outport
  wires:
  Schlauchparameter/1 -> Bus Creator5/2  "Tube"
  Bus Creator5/1 -> Signal Conversion/1  "Parameters"
  Wirksame Massen/1 -> min 50g/1
  Umgebungsdruck/1 -> Bus Creator4/1  "pAmb"
  Initiale Balglänge/1 -> Bus Creator3/1  "lBss"
  Wirksame Fläche (Druck)/1 -> Bus Creator3/4  "AP"
  Bus Creator3/1 -> Bus Creator5/4  "Bellows"
  Initialvolumen/1 -> Bus Creator3/2  "V0B"
  Steifigkeitsparameter Balg (p->l)/1 -> Bus Creator3/7  "ks_p2l_bar2m"
  min 50g/1 -> Bus Creator3/5  "MB"
  Wirksame Dämpfung/1 -> Bus Creator3/6  "dB"
  Dichte von Luft (Raumtemperatur)/1 -> Bus Creator4/4  "rho"
  Temperatur (Umgebung)/1 -> Bus Creator4/7  "T"
  Idealer Entlüftungsdruck/1 -> Bus Creator4/3  "pLow"
  Wirksame Fläche (Volumen)/1 -> Bus Creator3/3  "AV"
  Polytropenkoeffizient/1 -> Bus Creator4/5  "nK"
  Allg. Gaskonstante/1 -> Bus Creator4/6  "R"
  Steifigkeitsparameter Balg (l->b)/1 -> Bus Creator3/8  "ks_l2p_m2Pa"
  Bus Creator4/1 -> Bus Creator5/3  "Pressure"
  Signal Conversion/1 -> Parameters/1
  Idealer Belüftungsdruck/1 -> Bus Creator4/2  "pHigh"
  Max. Balgdruck/1 -> Bus Creator3/9  "pMax"
  Min. Balgdruck/1 -> Bus Creator3/10  "pMin"
  Max. Balglänge/1 -> Bus Creator3/11  "lB_max"
  Min. Balglänge/1 -> Bus Creator3/12  "lB_min"
  CInv: Flow-Chain-Factor/1 -> Bus Creator1/4  "cinv-fcf"
  CInv: Steigung M1/1 -> Bus Creator1/5  "cinv-m1"
  CInv: Steigung M2/1 -> Bus Creator1/6  "cinv-m2"
  CInv: Überdeckung/1 -> Bus Creator1/7  "cinv-xue"
  CInv: Ausrundung/1 -> Bus Creator1/8  "cinv-rund"
  CInv: Leckstrom/1 -> Bus Creator1/9  "cinv-leck"
  Cmax (Entlüften)/1 -> Bus Creator1/2  "Cmax-ent"
  Cmax (Belüften)/1 -> Bus Creator1/1  "Cmax-bel"
  Bus Creator1/1 -> Bus Creator5/1  "Valve"
  Kritischse Druckverhältnis b (MW)/1 -> Bus Creator1/3  "b-mean"
  CInv: Absenkung/1 -> Bus Creator1/12  "cinv-absk"
  CInv: Formparameter/1 -> Bus Creator1/13  "cinv-shape"
  CInv: Ausdellung/1 -> Bus Creator1/10  "cinv-delle"
  CInv: Zweite Überdeckung/1 -> Bus Creator1/11  "cinv-xue2"

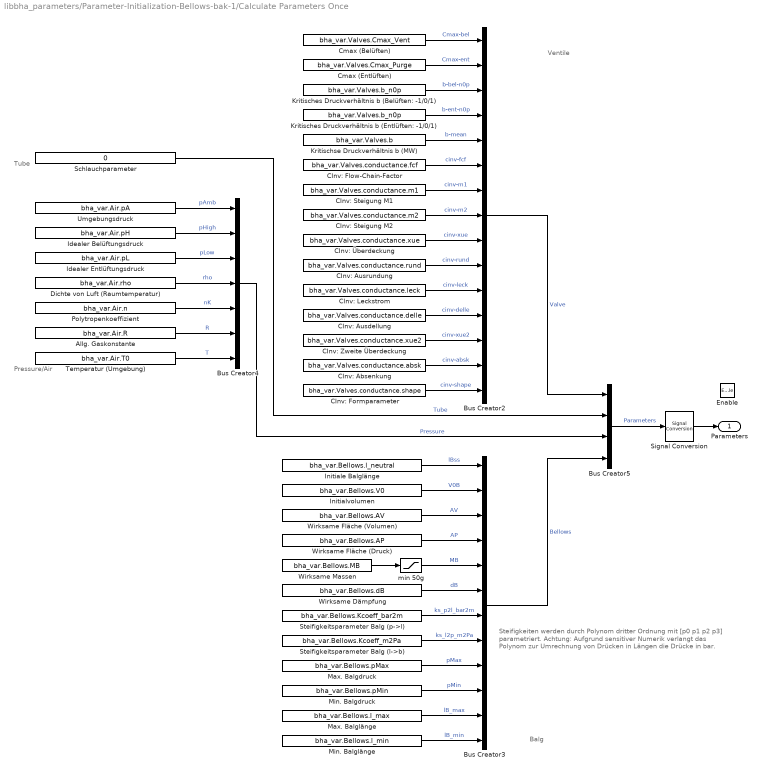
== system libbha_parameters/Parameter-Initialization-Bellows-bak-1/Calculate Parameters Once ==
  note: Ventile
  note: Steifigkeiten werden durch Polynom dritter Ordnung mit [p0 p1 p2 p3]
      | parametriert. Achtung: Aufgrund sensitiver Numerik verlangt das Polynom
      | zur Umrechnung von Drücken in Längen die Drücke in bar.
  note: Balg
  note: Pressure/Air
  note: Tube
  Enable : EnablePort  PropagateVarSize=During execution
  Allg. Gaskonstante : Constant  Value=bha_var.Air.R
  Bus Creator3 : BusCreator  Inputs=12
  Bus Creator4 : BusCreator  Inputs=7
  Bus Creator2 : BusCreator  Inputs=15
  Bus Creator5 : BusCreator  Inputs=4
  CInv: Absenkung : Constant  Value=bha_var.Valves.conductance.absk
  CInv: Ausdellung : Constant  Value=bha_var.Valves.conductance.delle
  CInv: Ausrundung : Constant  Value=bha_var.Valves.conductance.rund
  CInv: Flow-Chain-Factor : Constant  Value=bha_var.Valves.conductance.fcf
  CInv: Formparameter : Constant  Value=bha_var.Valves.conductance.shape
  CInv: Leckstrom : Constant  Value=bha_var.Valves.conductance.leck
  CInv: Steigung M1 : Constant  Value=bha_var.Valves.conductance.m1
  CInv: Steigung M2 : Constant  Value=bha_var.Valves.conductance.m2
  CInv: Zweite Überdeckung : Constant  Value=bha_var.Valves.conductance.xue2
  CInv: Überdeckung : Constant  Value=bha_var.Valves.conductance.xue
  Cmax (Belüften) : Constant  Value=bha_var.Valves.Cmax_Vent
  Cmax (Entlüften) : Constant  Value=bha_var.Valves.Cmax_Purge
  Dichte von Luft (Raumtemperatur) : Constant  Value=bha_var.Air.rho
  Idealer Belüftungsdruck : Constant  Value=bha_var.Air.pH
  Idealer Entlüftungsdruck : Constant  Value=bha_var.Air.pL
  Initiale Balglänge : Constant  Value=bha_var.Bellows.l_neutral
  Initialvolumen : Constant  Value=bha_var.Bellows.V0
  Kritisches Druckverhältnis b (Belüften: -1/0/1) : Constant  Value=bha_var.Valves.b_n0p
  Kritisches Druckverhältnis b (Entlüften: -1/0/1) : Constant  Value=bha_var.Valves.b_n0p
  Kritischse Druckverhältnis b (MW) : Constant  Value=bha_var.Valves.b
  Max. Balgdruck : Constant  Value=bha_var.Bellows.pMax
  Max. Balglänge : Constant  Value=bha_var.Bellows.l_max
  Min. Balgdruck : Constant  Value=bha_var.Bellows.pMin
  Min. Balglänge : Constant  Value=bha_var.Bellows.l_min
  Polytropenkoeffizient : Constant  Value=bha_var.Air.n
  Schlauchparameter : Constant  Value=0
  Signal Conversion : SignalConversion
  Steifigkeitsparameter Balg (l->b) : Constant  Value=bha_var.Bellows.Kcoeff_m2Pa
  Steifigkeitsparameter Balg (p->l) : Constant  Value=bha_var.Bellows.Kcoeff_bar2m
  Temperatur (Umgebung) : Constant  Value=bha_var.Air.T0
  Umgebungsdruck : Constant  Value=bha_var.Air.pA
  Wirksame Dämpfung : Constant  Value=bha_var.Bellows.dB
  Wirksame Fläche (Druck) : Constant  Value=bha_var.Bellows.AP
  Wirksame Fläche (Volumen) : Constant  Value=bha_var.Bellows.AV
  Wirksame Massen : Constant  Value=bha_var.Bellows.MB
  min 50g : Saturate  UpperLimit=inf  LowerLimit=0.1
  Parameters : Outport
  wires:
  CInv: Zweite Überdeckung/1 -> Bus Creator2/13  "cinv-xue2"
  CInv: Ausdellung/1 -> Bus Creator2/12  "cinv-delle"
  CInv: Formparameter/1 -> Bus Creator2/15  "cinv-shape"
  CInv: Absenkung/1 -> Bus Creator2/14  "cinv-absk"
  Kritischse Druckverhältnis b (MW)/1 -> Bus Creator2/5  "b-mean"
  Bus Creator2/1 -> Bus Creator5/1  "Valve"
  Kritisches Druckverhältnis b (Belüften: -1/0/1)/1 -> Bus Creator2/3  "b-bel-n0p"
  Cmax (Belüften)/1 -> Bus Creator2/1  "Cmax-bel"
  Cmax (Entlüften)/1 -> Bus Creator2/2  "Cmax-ent"
  Kritisches Druckverhältnis b (Entlüften: -1/0/1)/1 -> Bus Creator2/4  "b-ent-n0p"
  CInv: Leckstrom/1 -> Bus Creator2/11  "cinv-leck"
  CInv: Ausrundung/1 -> Bus Creator2/10  "cinv-rund"
  CInv: Überdeckung/1 -> Bus Creator2/9  "cinv-xue"
  CInv: Steigung M2/1 -> Bus Creator2/8  "cinv-m2"
  CInv: Steigung M1/1 -> Bus Creator2/7  "cinv-m1"
  CInv: Flow-Chain-Factor/1 -> Bus Creator2/6  "cinv-fcf"
  Min. Balglänge/1 -> Bus Creator3/12  "lB_min"
  Max. Balglänge/1 -> Bus Creator3/11  "lB_max"
  Min. Balgdruck/1 -> Bus Creator3/10  "pMin"
  Max. Balgdruck/1 -> Bus Creator3/9  "pMax"
  Idealer Belüftungsdruck/1 -> Bus Creator4/2  "pHigh"
  Signal Conversion/1 -> Parameters/1
  Bus Creator4/1 -> Bus Creator5/3  "Pressure"
  Steifigkeitsparameter Balg (l->b)/1 -> Bus Creator3/8  "ks_l2p_m2Pa"
  Allg. Gaskonstante/1 -> Bus Creator4/6  "R"
  Polytropenkoeffizient/1 -> Bus Creator4/5  "nK"
  Wirksame Fläche (Volumen)/1 -> Bus Creator3/3  "AV"
  Idealer Entlüftungsdruck/1 -> Bus Creator4/3  "pLow"
  Temperatur (Umgebung)/1 -> Bus Creator4/7  "T"
  Dichte von Luft (Raumtemperatur)/1 -> Bus Creator4/4  "rho"
  Wirksame Dämpfung/1 -> Bus Creator3/6  "dB"
  min 50g/1 -> Bus Creator3/5  "MB"
  Steifigkeitsparameter Balg (p->l)/1 -> Bus Creator3/7  "ks_p2l_bar2m"
  Initialvolumen/1 -> Bus Creator3/2  "V0B"
  Bus Creator3/1 -> Bus Creator5/4  "Bellows"
  Wirksame Fläche (Druck)/1 -> Bus Creator3/4  "AP"
  Initiale Balglänge/1 -> Bus Creator3/1  "lBss"
  Umgebungsdruck/1 -> Bus Creator4/1  "pAmb"
  Wirksame Massen/1 -> min 50g/1
  Bus Creator5/1 -> Signal Conversion/1  "Parameters"
  Schlauchparameter/1 -> Bus Creator5/2  "Tube"

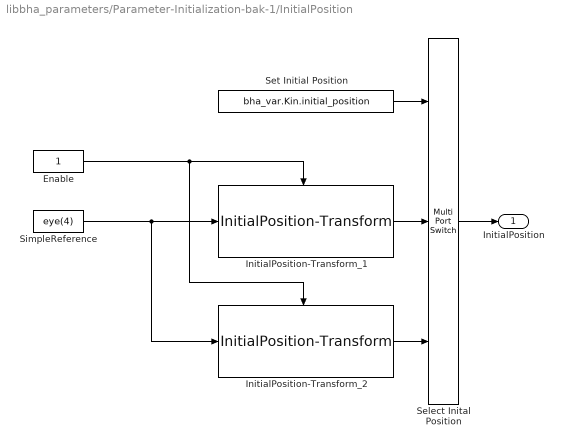
== system libbha_parameters/Parameter-Initialization-bak-1/InitialPosition ==
  Enable : Constant
  InitialPosition-Transform_1 : libbha_kinematic/InitialPosition-Transform  transx=bha_var.Kin.initial_translation(1)  transy=bha_var.Kin.initial_translation(2)  transz=bha_var.Kin.initial_translation(3)  positioning=Hängend  rotz=bha_var.Kin.initial_rotation
  InitialPosition-Transform_2 : libbha_kinematic/InitialPosition-Transform  transx=bha_var.Kin.initial_translation(1)  transy=bha_var.Kin.initial_translation(2)  transz=bha_var.Kin.initial_translation(3)  positioning=Stehend  rotz=bha_var.Kin.initial_rotation
  Select Inital Position : MultiPortSwitch  Inputs=2  DiagnosticForDefault=Warning
  Set Initial Position : Constant  Value=bha_var.Kin.initial_position
  SimpleReference : Constant  Value=eye(4)
  InitialPosition : Outport
  wires:
  Select Inital Position/1 -> InitialPosition/1
  Set Initial Position/1 -> Select Inital Position/1
  SimpleReference/1 -> InitialPosition-Transform_2/1, InitialPosition-Transform_1/1
  InitialPosition-Transform_1/1 -> Select Inital Position/2
  InitialPosition-Transform_2/1 -> Select Inital Position/3
  Enable/1 -> InitialPosition-Transform_2/Enable, InitialPosition-Transform_1/Enable

== system libbha_parameters/Parameter-Initialization-bak-1/ToolSetup ==
  Enable : Constant  Value=bha_var.Kin.VG_dx  SampleTime=CONST.tA
  Enable1 : Constant  Value=bha_var.Kin.VG_dz  SampleTime=CONST.tA
  Enable2 : Constant  Value=bha_var.Kin.VG_phiy  SampleTime=CONST.tA
  VacuumGripper_Tool : libbha_kinematic/VacuumGripper_Tool
  ToolSetup : Outport
  wires:
  VacuumGripper_Tool/1 -> ToolSetup/1
  Enable/1 -> VacuumGripper_Tool/1
  Enable2/1 -> VacuumGripper_Tool/3
  Enable1/1 -> VacuumGripper_Tool/2

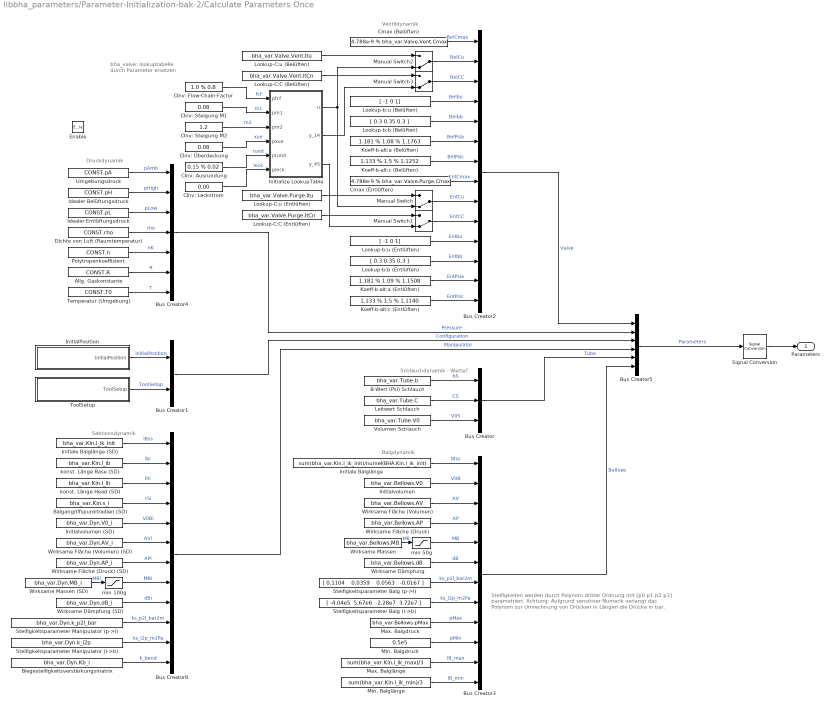
== system libbha_parameters/Parameter-Initialization-bak-2/Calculate Parameters Once ==
  note: Sektionsdynamik
  note: Ventildynamik
  note: Druckdynamik
  note: Balgdynamik
  note: Schlauchdynamik - Werte?
  note: Steifigkeiten werden durch Polynom dritter Ordnung mit [p0 p1 p2 p3]
      | parametriert. Achtung: Aufgrund sensitiver Numerik verlangt das Polynom
      | zur Umrechnung von Drücken in Längen die Drücke in bar.
  note: bha_valve: lookuptabelle
      | durch Parameter ersetzen
  Enable : EnablePort  PropagateVarSize=During execution
  Allg. Gaskonstante : Constant  Value=CONST.R
  B-Wert (Psi) Schlauch : Constant  Value=bha_var.Tube.b
  Balgangriffspunktradien (SD) : Constant  Value=bha_var.Kin.s_i
  Biegesteifigkeitsverstärkungsmatrix : Constant  Value=bha_var.Dyn.Kb_i
  Bus Creator1 : BusCreator  Inputs=2
  Bus Creator3 : BusCreator  Inputs=12
  Bus Creator4 : BusCreator  Inputs=7
  Bus Creator8 : BusCreator  Inputs=12
  Bus Creator : BusCreator  Inputs=3
  Bus Creator2 : BusCreator  Inputs=14
  Bus Creator5 : BusCreator  Inputs=6
  CInv: Ausrundung : Constant  Value=0.15 % 0.02
  CInv: Flow-Chain-Factor : Constant  Value=1.0 % 0.8
  CInv: Leckstrom : Constant  Value=0.00
  CInv: Steigung M1 : Constant  Value=0.08
  CInv: Steigung M2 : Constant  Value=1.2
  CInv: Überdeckung : Constant  Value=0.08
  Cmax (Belüften) : Constant  Value=4.788e-9 % bha_var.Valve.Vent.Cmax
  Cmax (Entlüften) : Constant  Value=4.788e-9 % bha_var.Valve.Purge.Cmax
  Dichte von Luft (Raumtemperatur) : Constant  Value=CONST.rho
  Idealer Belüftungsdruck : Constant  Value=CONST.pH
  Idealer Entlüftungsdruck : Constant  Value=CONST.pL
  InitialPosition : Subsystem
  Initiale Balglänge : Constant  Value=sum(bha_var.Kin.l_ik_init)/numel(BHA.Kin.l_ik_init)
  Initiale Balglänge (SD) : Constant  Value=bha_var.Kin.l_ik_init
  Initialize LookupTable : MATLAB Function  TreatAsAtomicUnit=on
  Initialvolumen : Constant  Value=bha_var.Bellows.V0
  Initialvolumen (SD) : Constant  Value=bha_var.Dyn.V0_i
  Koeff-b-alt:a (Belüften) : Constant  Value=1.181 % 1.08 % 1.1763
  Koeff-b-alt:a (Entlüften) : Constant  Value=1.181 % 1.09 % 1.1508
  Koeff-b-alt:c (Belüften) : Constant  Value=1.133 % 1.5 % 1.1252
  Koeff-b-alt:c (Entlüften) : Constant  Value=1.133 % 1.5 % 1.1140
  Leitwert Schlauch : Constant  Value=bha_var.Tube.C
  Lookup-C:C (Belüften) : Constant  Value=bha_var.Valve.Vent.ltCn
  Lookup-C:C (Entlüften) : Constant  Value=bha_var.Valve.Purge.ltCn
  Lookup-C:u (Belüften) : Constant  Value=bha_var.Valve.Vent.ltu
  Lookup-C:u (Entlüften) : Constant  Value=bha_var.Valve.Purge.ltu
  Lookup-b:b (Belüften) : Constant  Value=[ 0.3 0.35 0.3 ]
  Lookup-b:b (Entlüften) : Constant  Value=[ 0.3 0.35 0.3 ]
  Lookup-b:u (Belüften) : Constant  Value=[ -1 0 1]
  Lookup-b:u (Entlüften) : Constant  Value=[ -1 0 1]
  Manual Switch{,1..3} (4 alike) : ManualSwitch  CurrentSetting=0
  Max. Balgdruck : Constant  Value=bha_var.Bellows.pMax
  Max. Balglänge : Constant  Value=sum(bha_var.Kin.l_ik_max)/3
  Min. Balgdruck : Constant  Value=0.5e5
  Min. Balglänge : Constant  Value=sum(bha_var.Kin.l_ik_min)/3
  Polytropenkoeffizient : Constant  Value=CONST.n
  Signal Conversion : SignalConversion
  Steifigkeitsparameter Balg (l->b) : Constant  Value="[ -4.04e5  5.67e6  -2.28e7  3.72e7 ]"
  Steifigkeitsparameter Balg (p->l) : Constant  Value="[ 0.1104    0.0359    0.0563   -0.0167 ]"
  Steifigkeitsparameter Manipulator (l->b) : Constant  Value=bha_var.Dyn.k_l2p
  Steifigkeitsparameter Manipulator (p->l) : Constant  Value=bha_var.Dyn.k_p2l_bar
  Temperatur (Umgebung) : Constant  Value=CONST.T0
  ToolSetup : Subsystem
  Umgebungsdruck : Constant  Value=CONST.pA
  Volumen Schlauch : Constant  Value=bha_var.Tube.V0
  Wirksame Dämpfung : Constant  Value=bha_var.Bellows.dB
  Wirksame Dämpfung (SD) : Constant  Value=bha_var.Dyn.dB_i
  Wirksame Fläche (Druck) : Constant  Value=bha_var.Bellows.AP
  Wirksame Fläche (Druck) (SD) : Constant  Value=bha_var.Dyn.AP_i
  Wirksame Fläche (Volumen) : Constant  Value=bha_var.Bellows.AV
  Wirksame Fläche (Volumen) (SD) : Constant  Value=bha_var.Dyn.AV_i
  Wirksame Massen : Constant  Value=bha_var.Bellows.MB
  Wirksame Massen (SD) : Constant  Value=bha_var.Dyn.MB_i
  konst. Länge Base (SD) : Constant  Value=bha_var.Kin.l_ib
  konst. Länge Head (SD) : Constant  Value=bha_var.Kin.l_ih
  min 100g : Saturate  UpperLimit=inf  LowerLimit=0.1
  min 50g : Saturate  UpperLimit=inf  LowerLimit=0.1
  Parameters : Outport
  wires:
  Biegesteifigkeitsverstärkungsmatrix/1 -> Bus Creator8/12  "k_bend"
  Steifigkeitsparameter Manipulator (p->l)/1 -> Bus Creator8/10  "ks_p2l_bar2m"
  Steifigkeitsparameter Manipulator (l->b)/1 -> Bus Creator8/11  "ks_l2p_m2Pa"
  Bus Creator5/1 -> Signal Conversion/1  "Parameters"
  Wirksame Massen/1 -> min 50g/1  "MB"
  Wirksame Massen (SD)/1 -> min 100g/1  "MBi"
  Umgebungsdruck/1 -> Bus Creator4/1  "pAmb"
  Initiale Balglänge/1 -> Bus Creator3/1  "lBss"
  Wirksame Fläche (Druck)/1 -> Bus Creator3/4  "AP"
  B-Wert (Psi) Schlauch/1 -> Bus Creator/1  "bS"
  Volumen Schlauch/1 -> Bus Creator/3  "V0S"
  Leitwert Schlauch/1 -> Bus Creator/2  "CS"
  Bus Creator/1 -> Bus Creator5/5  "Tube"
  Bus Creator8/1 -> Bus Creator5/4  "Manipulator"
  min 100g/1 -> Bus Creator8/8  "MBi"
  Bus Creator3/1 -> Bus Creator5/6  "Bellows"
  Initialvolumen (SD)/1 -> Bus Creator8/5  "V0Bi"
  Wirksame Dämpfung (SD)/1 -> Bus Creator8/9  "dBi"
  ToolSetup/1(ToolSetup) -> Bus Creator1/2  "ToolSetup"
  Wirksame Fläche (Druck) (SD)/1 -> Bus Creator8/7  "APi"
  Wirksame Fläche (Volumen) (SD)/1 -> Bus Creator8/6  "AVi"
  Initialvolumen/1 -> Bus Creator3/2  "V0B"
  Steifigkeitsparameter Balg (p->l)/1 -> Bus Creator3/7  "ks_p2l_bar2m"
  konst. Länge Head (SD)/1 -> Bus Creator8/3  "lhi"
  konst. Länge Base (SD)/1 -> Bus Creator8/2  "lbi"
  Balgangriffspunktradien (SD)/1 -> Bus Creator8/4  "rSi"
  min 50g/1 -> Bus Creator3/5  "MB"
  Wirksame Dämpfung/1 -> Bus Creator3/6  "dB"
  Dichte von Luft (Raumtemperatur)/1 -> Bus Creator4/4  "rho"
  Temperatur (Umgebung)/1 -> Bus Creator4/7  "T"
  Idealer Entlüftungsdruck/1 -> Bus Creator4/3  "pLow"
  Wirksame Fläche (Volumen)/1 -> Bus Creator3/3  "AV"
  Bus Creator2/1 -> Bus Creator5/1  "Valve"
  Polytropenkoeffizient/1 -> Bus Creator4/5  "nK"
  Allg. Gaskonstante/1 -> Bus Creator4/6  "R"
  InitialPosition/1(InitialPosition) -> Bus Creator1/1  "InitialPosition"
  Steifigkeitsparameter Balg (l->b)/1 -> Bus Creator3/8  "ks_l2p_m2Pa"
  Bus Creator4/1 -> Bus Creator5/2  "Pressure"
  Initiale Balglänge (SD)/1 -> Bus Creator8/1  "lBss"
  Bus Creator1/1 -> Bus Creator5/3  "Configuration"
  Signal Conversion/1 -> Parameters/1
  Idealer Belüftungsdruck/1 -> Bus Creator4/2  "pHigh"
  Lookup-b:b (Belüften)/1 -> Bus Creator2/5  "Belbb"
  Cmax (Belüften)/1 -> Bus Creator2/1  "BelCmax"
  Koeff-b-alt:a (Belüften)/1 -> Bus Creator2/6  "BelPsia"
  Koeff-b-alt:c (Belüften)/1 -> Bus Creator2/7  "BelPsic"
  Lookup-b:u (Belüften)/1 -> Bus Creator2/4  "Belbu"
  Manual Switch3/1 -> Bus Creator2/3  "BelCC"
  Manual Switch2/1 -> Bus Creator2/2  "BelCu"
  Cmax (Entlüften)/1 -> Bus Creator2/8  "EntCmax"
  Manual Switch1/1 -> Bus Creator2/10  "EntCC"
  Manual Switch/1 -> Bus Creator2/9  "EntCu"
  Lookup-b:b (Entlüften)/1 -> Bus Creator2/12  "Entbb"
  Lookup-b:u (Entlüften)/1 -> Bus Creator2/11  "Entbu"
  Koeff-b-alt:a (Entlüften)/1 -> Bus Creator2/13  "EntPsia"
  Koeff-b-alt:c (Entlüften)/1 -> Bus Creator2/14  "EntPsic"
  Initialize LookupTable/1(u) -> Manual Switch/2, Manual Switch2/2
  Initialize LookupTable/2(y_14) -> Manual Switch3/2
  Initialize LookupTable/3(y_45) -> Manual Switch1/2
  Lookup-C:C (Entlüften)/1 -> Manual Switch1/1
  Lookup-C:u (Entlüften)/1 -> Manual Switch/1
  Lookup-C:u (Belüften)/1 -> Manual Switch2/1
  Lookup-C:C (Belüften)/1 -> Manual Switch3/1
  CInv: Leckstrom/1 -> Initialize LookupTable/6(pleck)  "leck"
  CInv: Ausrundung/1 -> Initialize LookupTable/5(prund)  "rund"
  CInv: Überdeckung/1 -> Initialize LookupTable/4(pxue)  "xue"
  CInv: Steigung M2/1 -> Initialize LookupTable/3(pm2)  "m2"
  CInv: Steigung M1/1 -> Initialize LookupTable/2(pm1)  "m1"
  CInv: Flow-Chain-Factor/1 -> Initialize LookupTable/1(pfcf)  "fcf"
  Max. Balgdruck/1 -> Bus Creator3/9  "pMax"
  Min. Balgdruck/1 -> Bus Creator3/10  "pMin"
  Max. Balglänge/1 -> Bus Creator3/11  "lB_max"
  Min. Balglänge/1 -> Bus Creator3/12  "lB_min"
